simulink model "Final_PV2"  (R2017a)
settings: Solver=ode45  StartTime=0.0  StopTime=10  MinStep=.00000001  RelTol=1e-7  EnableMultiTasking=on
libraries: powerlib x8, simulink x2
settings Model: Creator=TCM  LastModifiedBy=Kimo Store
settings SolverCC: ZeroCrossControl=EnableAll  AlgebraicLoopSolver=LineSearch
settings DataIOCC: LimitDataPoints=on  SaveFormat=Array
settings OptimizationCC: LifeSpan=inf
settings DebuggingCC: UnderspecifiedInitializationDetection=Classic  MergeDetectMultiDrivingBlocksExec=none  SolverPrmCheckMsg=warning  StateNameClashWarn=warning  SFUnexpectedBacktrackingDiag=warning  SFNoUnconditionalDefaultTransitionDiag=warning  SFExecutionAtInitializationDiag=none
settings HardwareCC: ProdBitPerPointer=32  ProdBitPerSizeT=32  ProdBitPerPtrDiffT=32  ProdLargestAtomicFloat=None  ProdIntDivRoundTo=Undefined  ProdEndianess=Unspecified  ProdWordSize=32  ProdHWDeviceType=32-bit Generic
settings ModelReferenceCC: PropagateSignalLabelsOutOfModel=off
settings GRTTargetCC: TargetLangStandard=C89/C90 (ANSI)  GeneratePreprocessorConditionals=Disable all
settings ConfigComp: CovMetricSettings=dw  CovHtmlReporting=on  CovSaveCumulativeToWorkspaceVar=on  CovSaveSingleToWorkspaceVar=on  CovExternalEMLEnable=off

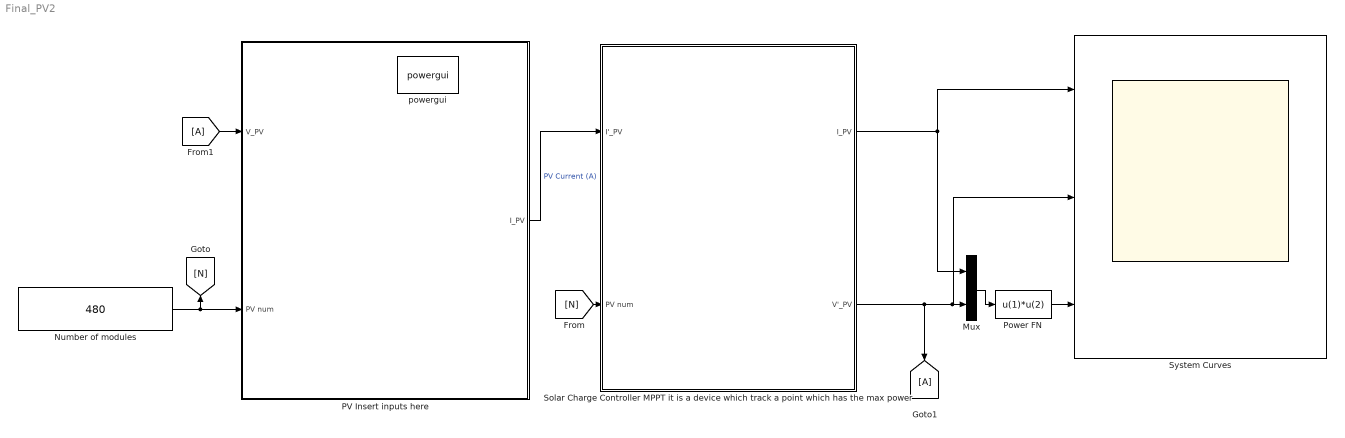
== system Final_PV2 ==
  Mux : Mux  Inputs=2
  Number of modules : Constant  Value=480
  PV Insert inputs here : Subsystem
      mask Display: image('C:\Users\Kimo Store\Desktop\PV Simulink\pva.jpg');
  "Power FN " : Fcn  Expr=u(1)*u(2)
  Solar Charge Controller MPPT it is a device which track a point which has the max power : Subsystem
  System Curves : Scope  NumInputPorts=3
  powergui : powerlib/powergui  Priority=1  SimulationMode=Continuous  SampleTime=50e-6  frequency=60  Iterations=50  frequencyindice=0  Pbase=100e6  ErrMax=1e-4  UnitsV=kV  UnitsW=MW  buscounter=0  FunctionMessages=off  echomessages=off  EnableUseOfTLC=off  CurrentSourceSwitches=off  DisableSnubberDevices=off  DisableRonSwitches=off  DisableVfSwitches=off  DisplayEquations=off  SolverType=Tustin  Interpol=off  ExternalGateDelay=off  methode=off  Ts=100  x0status=blocks  SPID=on  SwTol=0  HookPort=off  RestoreLinks=warning  ResistiveCurrentMeasurement=off  Frange=[0:2:500]  Ylog=off  Xlog=on  ShowGrid=off  save=off  variable=ZData  structure=0  ZoomFFT=off  StartTime=0.0  cycles=1  DisplayStyle=1  fundamental=60  FreqAxis=off  MaxFrequency=1000  frequencyindicesteady=1  RmsSteady=1  display=off
  wires:
  Number of modules/1 -> PV Insert inputs here/2(PV num), [N]
  [N] -> Solar Charge Controller MPPT it is a device which track a point which has the max power/2(PV num)
  Mux/1 -> "Power FN "/1
  "Power FN "/1 -> System Curves/3
  PV Insert inputs here/1(I_PV) -> Solar Charge Controller MPPT it is a device which track a point which has the max power/1(I'_PV)  "PV Current (A)"
  Solar Charge Controller MPPT it is a device which track a point which has the max power/2("V'_PV ") -> [A], System Curves/2, Mux/2
  [A] -> PV Insert inputs here/1(V_PV)
  Solar Charge Controller MPPT it is a device which track a point which has the max power/1(I_PV) -> Mux/1, System Curves/1

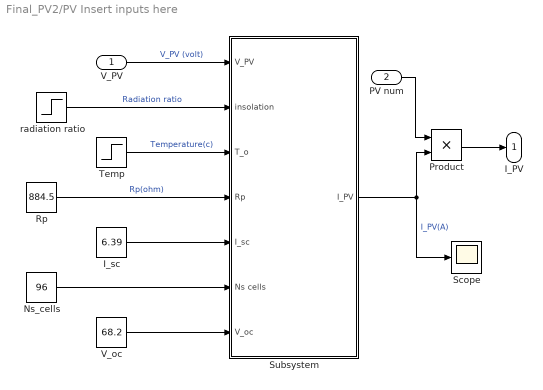
== system Final_PV2/PV Insert inputs here ==
  V_PV : Inport
  PV num : Inport  Port=2
  I_sc : Constant  Value=6.39
  Ns_cells : Constant  Value=96
  Product : Product
  Rp : Constant  Value=884.5
  Scope : Scope
  Subsystem : Subsystem
  Temp : Step  Time=5  Before=25  After=25  SampleTime=0
  V_oc : Constant  Value=68.2
  radiation ratio : Step  Before=1  SampleTime=0
  I_PV : Outport
  wires:
  Subsystem/1(I_PV) -> Scope/1, Product/2  "I_PV(A)"
  Temp/1 -> Subsystem/3(T_o)  "Temperature(c)"
  radiation ratio/1 -> Subsystem/2(insolation)  "Radiation ratio"
  Rp/1 -> Subsystem/4(Rp)  "Rp(ohm)"
  V_PV/1 -> Subsystem/1(V_PV)  "V_PV (volt)"
  Product/1 -> I_PV/1
  PV num/1 -> Product/1
  I_sc/1 -> Subsystem/5(I_sc)
  Ns_cells/1 -> Subsystem/6(Ns cells)
  V_oc/1 -> Subsystem/7(V_oc)

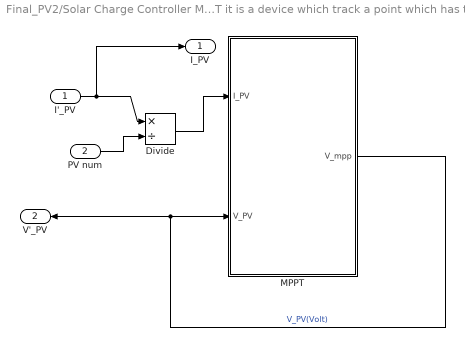
== system Final_PV2/Solar Charge Controller MPPT it is a device which track a point which has the max power ==
  I'_PV : Inport
  PV num : Inport  Port=2
  Divide : Product  Inputs=*/
  "MPPT " : Subsystem
  I_PV : Outport
  "V'_PV " : Outport  Port=2
  wires:
  "MPPT "/1(V_mpp) -> "V'_PV "/1, "MPPT "/2(V_PV)  "V_PV(Volt)"
  I'_PV/1 -> I_PV/1, Divide/1
  Divide/1 -> "MPPT "/1(I_PV)
  PV num/1 -> Divide/2

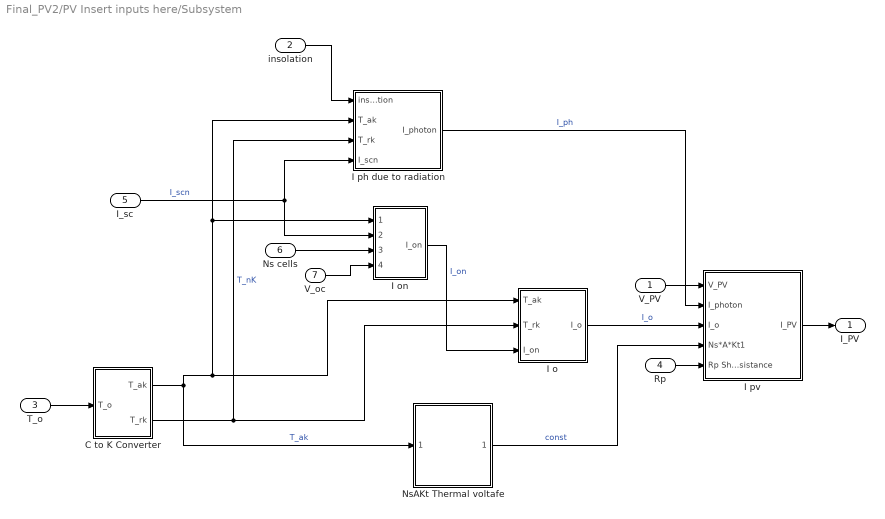
== system Final_PV2/PV Insert inputs here/Subsystem ==
  V_PV : Inport
  insolation : Inport  Port=2
  T_o : Inport  Port=3
  Rp : Inport  Port=4
  I_sc : Inport  Port=5
  Ns cells : Inport  Port=6
  V_oc : Inport  Port=7
  "C to K Converter " : Subsystem
  I o : Subsystem
  I on : Subsystem
  "I ph due to radiation " : Subsystem
  I pv : Subsystem
  NsAKt Thermal voltafe : Subsystem
  I_PV : Outport
  wires:
  T_o/1 -> "C to K Converter "/1(T_o)
  insolation/1 -> "I ph due to radiation "/1(insolation)
  "C to K Converter "/2(T_rk) -> I o/2(T_rk), "I ph due to radiation "/3(T_rk)  "T_nK"
  I_sc/1 -> "I ph due to radiation "/4(I_scn), I on/2(I_scn)  "I_scn"
  NsAKt Thermal voltafe/1(Ns*a*Kt) -> I pv/4(Ns*A*Kt1)  "const"
  I on/1(I_on) -> I o/3(I_on)  "I_on"
  "C to K Converter "/1(T_ak) -> "I ph due to radiation "/2(T_ak), I on/1(T_ref), I o/1(T_ak), NsAKt Thermal voltafe/1(T_ak T in kelven)  "T_ak"
  "I ph due to radiation "/1(I_photon) -> I pv/2(I_photon)  "I_ph"
  I pv/1(I_PV) -> I_PV/1
  I o/1(I_o) -> I pv/3(I_o)  "I_o"
  V_PV/1 -> I pv/1(V_PV)
  Rp/1 -> I pv/5(Rp Shunt resistance)
  Ns cells/1 -> I on/3(Num series)
  V_oc/1 -> I on/4(V_oc)

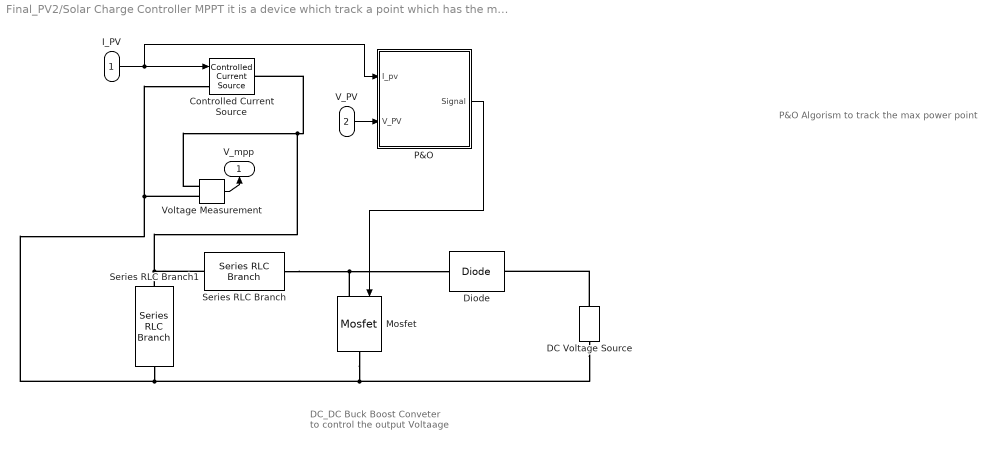
== system Final_PV2/Solar Charge Controller MPPT it is a device which track a point which has the max power/MPPT  ==
  note: P&O Algorism to track the max power point
  note: DC_DC Buck Boost Conveter
      |
      | to control the output Voltaage
  I_PV : Inport
  V_PV : Inport  Port=2
  Controlled Current Source : powerlib/Electrical Sources/Controlled Current Source  Initialize=on  Source_Type=DC  Amplitude=0  Phase=0  Frequency=0  Measurements=None
  DC Voltage Source : powerlib/Electrical Sources/DC Voltage Source  Amplitude=55  Measurements=None
  Diode : powerlib/Power Electronics/Diode  Ron=0.001  Lon=0  Vf=0.8  IC=0  UseSnubber=off  Rs=500  Cs=250e-9  Measurements=off
  Mosfet : powerlib/Power Electronics/Mosfet  Ron=0.001  Lon=0  Rd=0.01  Vfd=0  IC=0  Rs=1e5  Cs=inf  Measurements=off
  "P&O " : Subsystem
  Series RLC Branch : powerlib/Elements/Series RLC Branch  LConnTagsString=__new0  RConnTagsString=__new0  BranchType=RL  Resistance=.45  Inductance=1e-3  SetiL0=off  InitialCurrent=0  Capacitance=1e-6  Setx0=off  InitialVoltage=0  Measurements=None
  Series RLC Branch1 : powerlib/Elements/Series RLC Branch  LConnTagsString=__new0  RConnTagsString=__new0  BranchType=C  Resistance=1  Inductance=1e-3  SetiL0=off  InitialCurrent=0  Capacitance=2e-3  Setx0=off  InitialVoltage=0  Measurements=None
  Voltage Measurement : powerlib/Measurements/Voltage Measurement  PhasorSimulation=off  OutputType=Complex  PSBequivalent=0
  V_mpp : Outport
  wires:
  Voltage Measurement/1 -> V_mpp/1
  I_PV/1 -> "P&O "/1(I_pv), Controlled Current Source/1
  V_PV/1 -> "P&O "/2(V_PV)
  "P&O "/1(Signal) -> Mosfet/1
  connections:
  Series RLC Branch/RConn1 -- Mosfet/LConn1 -- Diode/LConn1
  Voltage Measurement/LConn1 -- Series RLC Branch/LConn1 -- Series RLC Branch1/LConn1 -- Controlled Current Source/RConn1
  Voltage Measurement/LConn2 -- DC Voltage Source/LConn1 -- Mosfet/RConn1 -- Series RLC Branch1/RConn1 -- Controlled Current Source/LConn1
  DC Voltage Source/RConn1 -- Diode/RConn1

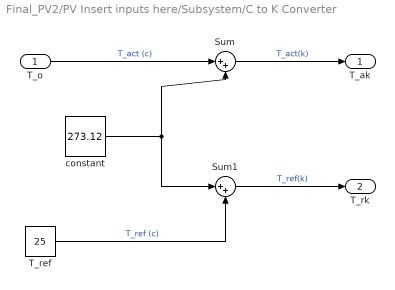
== system Final_PV2/PV Insert inputs here/Subsystem/C to K Converter  ==
  T_o : Inport
  Sum : Sum  Inputs=|++
  Sum1 : Sum  Inputs=|++
  T_ref : Constant  Value=25
  constant : Constant  Value=273.12
  T_ak : Outport
  T_rk : Outport  Port=2
  wires:
  constant/1 -> Sum1/1, Sum/2
  T_o/1 -> Sum/1  "T_act (c)"
  T_ref/1 -> Sum1/2  "T_ref (c)"
  Sum/1 -> T_ak/1  "T_act(k)"
  Sum1/1 -> T_rk/1  "T_ref(k)"

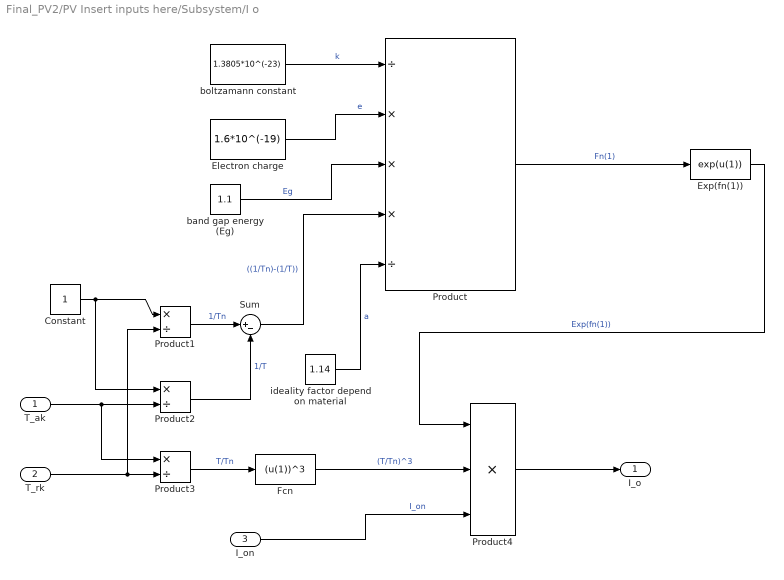
== system Final_PV2/PV Insert inputs here/Subsystem/I o ==
  T_ak : Inport
  T_rk : Inport  Port=2
  I_on : Inport  Port=3
  Constant : Constant
  Electron charge : Constant  Value=1.6*10^(-19)
  Exp(fn(1)) : Fcn  Expr=exp(u(1))
  Fcn : Fcn  Expr=(u(1))^3
  Product : Product  Inputs=/***/
  Product1 : Product  Inputs=*/
  Product2 : Product  Inputs=*/
  Product3 : Product  Inputs=*/
  Product4 : Product  Inputs=3
  Sum : Sum  Inputs=|+-
  band gap energy (Eg) : Constant  Value=1.1
  boltzamann constant : Constant  Value=1.3805*10^(-23)
  ideality factor depend on material : Constant  Value=1.14
  I_o : Outport
  wires:
  Electron charge/1 -> Product/2  "e"
  boltzamann constant/1 -> Product/1  "k"
  Product2/1 -> Sum/2  "1/T"
  I_on/1 -> Product4/3  "I_on"
  band gap energy (Eg)/1 -> Product/3  "Eg"
  Sum/1 -> Product/4  "((1/Tn)-(1/T))"
  Product3/1 -> Fcn/1  "T/Tn"
  Product1/1 -> Sum/1  "1/Tn"
  Constant/1 -> Product2/1, Product1/1
  ideality factor depend on material/1 -> Product/5  "a"
  T_ak/1 -> Product3/1, Product2/2
  Fcn/1 -> Product4/2  "(T/Tn)^3"
  Product/1 -> Exp(fn(1))/1  "Fn(1)"
  Exp(fn(1))/1 -> Product4/1  "Exp(fn(1))"
  T_rk/1 -> Product1/2, Product3/2
  Product4/1 -> I_o/1

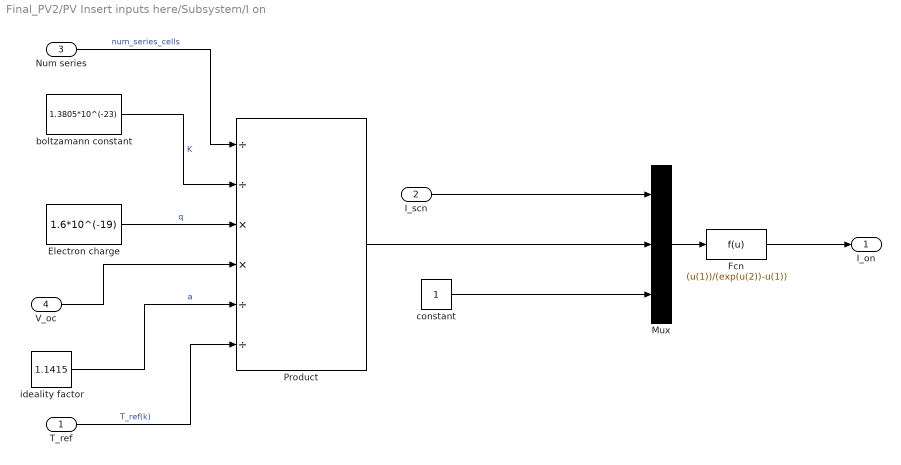
== system Final_PV2/PV Insert inputs here/Subsystem/I on ==
  T_ref : Inport
  I_scn : Inport  Port=2
  Num series : Inport  Port=3
  V_oc : Inport  Port=4
  Electron charge : Constant  Value=1.6*10^(-19)
  Fcn : Fcn  Expr=(u(1))/(exp(u(2))-u(1))
  Mux : Mux  Inputs=3
  Product : Product  Inputs=//**//
  boltzamann constant : Constant  Value=1.3805*10^(-23)
  constant : Constant
  ideality factor : Constant  Value=1.1415
  I_on : Outport
  wires:
  Num series/1 -> Product/1  "num_series_cells"
  boltzamann constant/1 -> Product/2  "K"
  Electron charge/1 -> Product/3  "q"
  ideality factor/1 -> Product/5  "a"
  T_ref/1 -> Product/6  "T_ref(k)"
  Product/1 -> Mux/2
  I_scn/1 -> Mux/1
  constant/1 -> Mux/3
  Mux/1 -> Fcn/1
  Fcn/1 -> I_on/1
  V_oc/1 -> Product/4

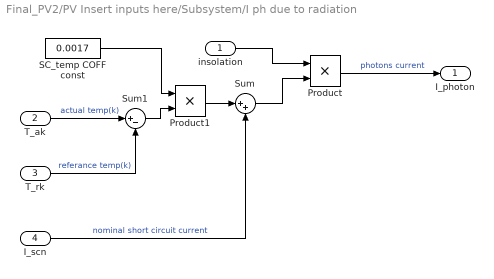
== system Final_PV2/PV Insert inputs here/Subsystem/I ph due to radiation  ==
  insolation : Inport
  T_ak : Inport  Port=2
  T_rk : Inport  Port=3
  I_scn : Inport  Port=4
  Product : Product
  Product1 : Product
  SC_temp COFF const : Constant  Value=0.0017
  Sum : Sum  Inputs=|++
  Sum1 : Sum  Inputs=|+-
  I_photon : Outport
  wires:
  Product/1 -> I_photon/1  "photons current"
  insolation/1 -> Product/1
  T_ak/1 -> Sum1/1  "actual temp(k)"
  T_rk/1 -> Sum1/2  "referance temp(k)"
  Sum/1 -> Product/2
  I_scn/1 -> Sum/2  "nominal short circuit current"
  Product1/1 -> Sum/1
  SC_temp COFF const/1 -> Product1/1
  Sum1/1 -> Product1/2

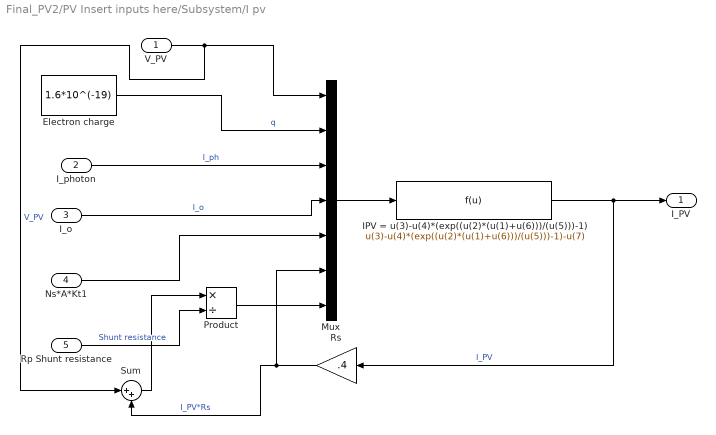
== system Final_PV2/PV Insert inputs here/Subsystem/I pv ==
  V_PV : Inport
  I_photon : Inport  Port=2
  I_o : Inport  Port=3
  Ns*A*Kt1 : Inport  Port=4
  Rp Shunt resistance : Inport  Port=5
  Electron charge : Constant  Value=1.6*10^(-19)
  IPV = u(3)-u(4)*(exp((u(2)*(u(1)+u(6)))/(u(5)))-1) : Fcn  Expr=u(3)-u(4)*(exp((u(2)*(u(1)+u(6)))/(u(5)))-1)-u(7)
  Mux : Mux  Inputs=7
  Product : Product  Inputs=*/
  Rs : Gain  Gain=.4
  Sum : Sum  Inputs=|++
  I_PV : Outport
  wires:
  IPV = u(3)-u(4)*(exp((u(2)*(u(1)+u(6)))/(u(5)))-1)/1 -> I_PV/1, Rs/1  "I_PV"
  Ns*A*Kt1/1 -> Mux/5
  Mux/1 -> IPV = u(3)-u(4)*(exp((u(2)*(u(1)+u(6)))/(u(5)))-1)/1
  I_o/1 -> Mux/4  "I_o"
  Rs/1 -> Sum/2, Mux/6  "I_PV*Rs"
  Electron charge/1 -> Mux/2  "q"
  I_photon/1 -> Mux/3  "I_ph"
  V_PV/1 -> Sum/1, Mux/1  "V_PV"
  Sum/1 -> Product/1
  Rp Shunt resistance/1 -> Product/2  "Shunt resistance"
  Product/1 -> Mux/7

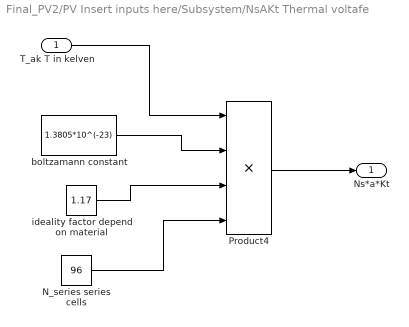
== system Final_PV2/PV Insert inputs here/Subsystem/NsAKt Thermal voltafe ==
  T_ak T in kelven : Inport
  N_series series cells : Constant  Value=96
  Product4 : Product  Inputs=4
  boltzamann constant : Constant  Value=1.3805*10^(-23)
  ideality factor depend on material : Constant  Value=1.17
  Ns*a*Kt : Outport
  wires:
  Product4/1 -> Ns*a*Kt/1
  boltzamann constant/1 -> Product4/2
  ideality factor depend on material/1 -> Product4/3
  T_ak T in kelven/1 -> Product4/1
  N_series series cells/1 -> Product4/4

== system Final_PV2/Solar Charge Controller MPPT it is a device which track a point which has the max power/MPPT /P&O  ==
  I_pv : Inport
  V_PV : Inport  Port=2
  P & O : Subsystem
  Saturation : Saturate  UpperLimit=1
  Subsystem1 : Subsystem
  Signal : Outport
  wires:
  P & O/1(signal) -> Saturation/1
  V_PV/1 -> P & O/2(Vpv)
  Saturation/1 -> Subsystem1/1(In1)
  Subsystem1/1(Out1) -> Signal/1
  I_pv/1 -> P & O/1(Ipv)

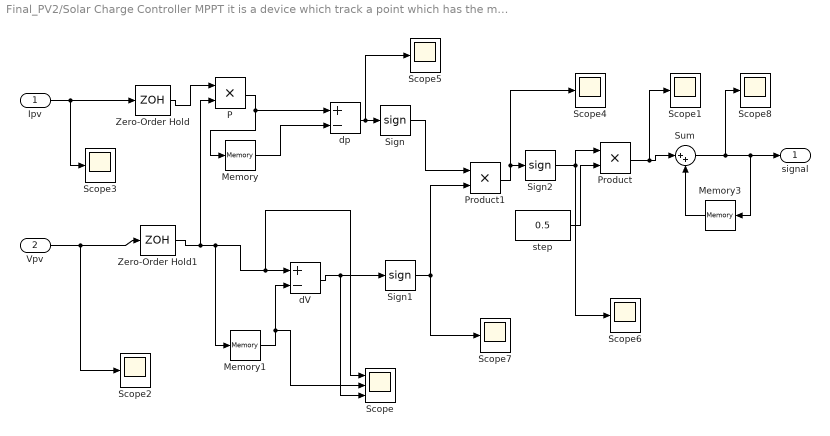
== system Final_PV2/Solar Charge Controller MPPT it is a device which track a point which has the max power/MPPT /P&O /P & O ==
  Ipv : Inport
  Vpv : Inport  Port=2
  Memory : Memory  InheritSampleTime=on
  Memory1 : Memory  InheritSampleTime=on
  Memory3 : Memory  InheritSampleTime=on
  P : Product  RndMeth=Zero
  Product : Product  RndMeth=Zero
  Product1 : Product  RndMeth=Zero
  Scope : Scope  NumInputPorts=3
  Scope{1..8} (8 alike) : Scope
  Sign : Signum
  Sign1 : Signum
  Sign2 : Signum
  Sum : Sum  Inputs=|++
  Zero-Order Hold : ZeroOrderHold  SampleTime=0.002
  Zero-Order Hold1 : ZeroOrderHold  SampleTime=0.002
  dV : Sum  Inputs=+-
  dp : Sum  Inputs=+-
  step : Constant  Value=0.5
  signal : Outport
  wires:
  Memory1/1 -> dV/2, Scope/2
  Memory/1 -> dp/2
  Vpv/1 -> Zero-Order Hold1/1, Scope2/1
  dV/1 -> Sign1/1, Scope/3
  step/1 -> Product/2
  Product/1 -> Sum/1, Scope1/1
  Sign/1 -> Product1/1
  Sign1/1 -> Product1/2, Scope7/1
  Product1/1 -> Sign2/1, Scope4/1
  Ipv/1 -> Zero-Order Hold/1, Scope3/1
  Zero-Order Hold1/1 -> P/2, dV/1, Scope/1, Memory1/1
  Zero-Order Hold/1 -> P/1
  P/1 -> Memory/1, dp/1
  dp/1 -> Sign/1, Scope5/1
  Sign2/1 -> Product/1, Scope6/1
  Sum/1 -> Memory3/1, signal/1, Scope8/1
  Memory3/1 -> Sum/2

== system Final_PV2/Solar Charge Controller MPPT it is a device which track a point which has the max power/MPPT /P&O /Subsystem1 ==
  In1 : Inport
  Compare To Zero : simulink/Logic and Bit Operations/Compare To Zero  relop=<=  OutDataTypeStr=boolean
  Repeating Sequence : simulink/Sources/Repeating Sequence  rep_seq_t=[0 0.1e-3]  rep_seq_y=[0 1]
  Subtract : Sum  Inputs=+-
  Out1 : Outport
  wires:
  Subtract/1 -> Compare To Zero/1
  Repeating Sequence/1 -> Subtract/2
  In1/1 -> Subtract/1
  Compare To Zero/1 -> Out1/1
